simulink model "Lab2Videoblock"  (R2022a)
settings: Solver=VariableStepAuto  StartTime=0.0  StopTime=1  MaxStep=1e-4  RelTol=1e-3
undefined symbols (not defined in the file or in its folder): ACsource, Angle, DCsource, load, transparam
libraries: spsFourierLib x4, spsGroundLib x4, spsVoltageMeasurementLib x4, spsCurrentMeasurementLib x3, spsACVoltageSourceLib x1, spsDiodeLib x1, spsDCVoltageSourceLib x1, spsLinearTransformerLib x1, spsMultimeterLib x1, spsSeriesRLCBranchLib x1, spsRMSLib x1, spsUniversalBridgeLib x1
settings Model: Creator=Student11  LastModifiedBy=админ
settings SolverCC: AlgebraicLoopSolver=TrustRegion
settings DataIOCC: ReturnWorkspaceOutputs=off
settings DebuggingCC: SFMachineParentedDataDiag=warning  ArithmeticOperatorsInVariantConditions=warning
settings SFSimCC: SimUseLocalCustomCode=off  CustomCodeUndefinedFunction=UseInterfaceOnly
settings RTWCC: RTWUseLocalCustomCode=off
settings CodeAppCC: StateflowObjectComments=on
settings SimscapeCC: SimscapeNormalizeSystem=off

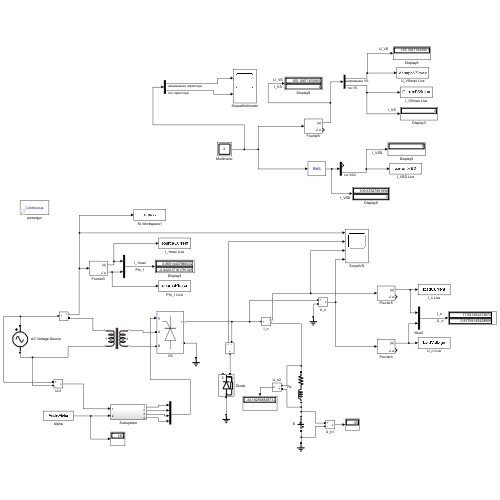
[thumbnail: Simulink's stored preview of the top-level diagram]
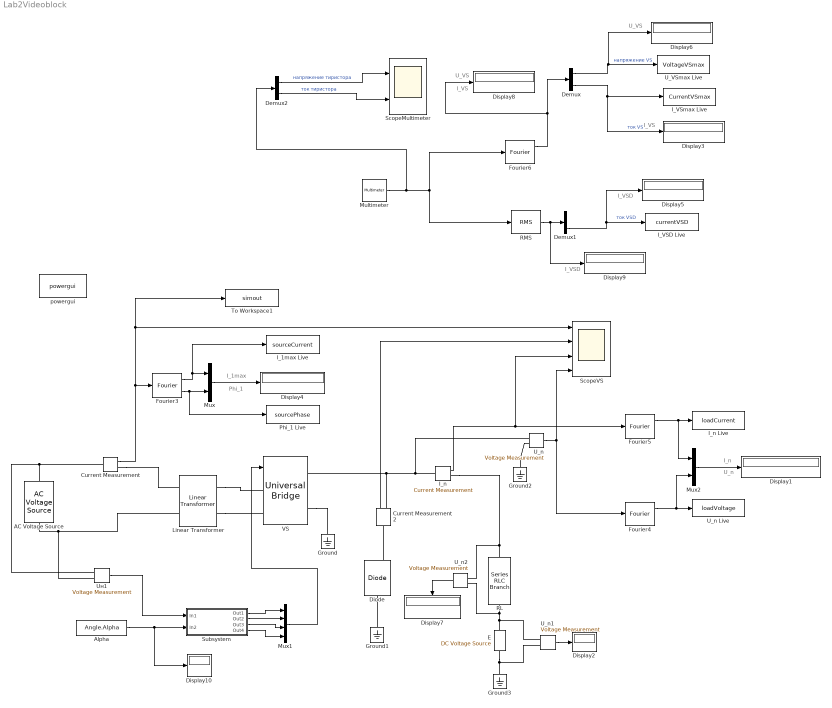
== system Lab2Videoblock ==
  note: U_VS
  note: I_VS
  note: I_VSD
  note: Phi_1
  note: I_1max
  note: I_n
  note: U_n
  note: I_VS
  note: U_VS
  note: I_VSD
  AC Voltage Source : spsACVoltageSourceLib/AC Voltage Source  Amplitude=ACsource.voltage  Phase=0  Frequency=ACsource.freq  SampleTime=0  Measurements=None  BusType=swing  Pref=10e3  Qref=0  Qmin=-inf  Qmax=+inf
  Alpha : Constant  Value=Angle.Alpha
  Current Measurement : spsCurrentMeasurementLib/Current Measurement  PhasorSimulation=off  OutputType=Complex  PSBequivalent=0
  Current Measurement2 : spsCurrentMeasurementLib/Current Measurement  PhasorSimulation=off  OutputType=Complex  PSBequivalent=0
  Demux : Demux  Outputs=2
  Demux1 : Demux  Outputs=2
  Demux2 : Demux  Outputs=2
  Diode : spsDiodeLib/Diode  Ron=0.001  Lon=0  Vf=0.8  IC=0  UseSnubber=0  Rs=500  Cs=250e-9  Measurements=on
  Display{1..10} (10 alike) : Display
      Display1 settings: Format=binary (Stored Integer)
      Display10 settings: Format=binary (Stored Integer)
      Display2 settings: Format=binary (Stored Integer)
      Display3 settings: Format=binary (Stored Integer)  Decimation=2
      Display4 settings: Format=binary (Stored Integer)  Decimation=2
      Display5 settings: Format=binary (Stored Integer)  Decimation=2
      Display6 settings: Format=binary (Stored Integer)  Decimation=2
      Display7 settings: Format=binary (Stored Integer)
      Display8 settings: Format=binary (Stored Integer)  Decimation=2
      Display9 settings: Format=binary (Stored Integer)  Decimation=2
  E : spsDCVoltageSourceLib/DC Voltage Source  Amplitude=DCsource.voltage  Measurements=None
  Fourier3 : spsFourierLib/Fourier  Freq=ACsource.freq  n=1  InInit=[0, 0]  Ts=0
      settings: SourceProductBaseCode=PS
  Fourier4 : spsFourierLib/Fourier  Freq=ACsource.freq  n=0  InInit=[0, 0]  Ts=0
      settings: SourceProductBaseCode=PS
  Fourier5 : spsFourierLib/Fourier  Freq=ACsource.freq  n=0  InInit=[0, 0]  Ts=0
      settings: SourceProductBaseCode=PS
  Fourier6 : spsFourierLib/Fourier  Freq=ACsource.freq  n=1  InInit=[0, 0]  Ts=0
      settings: SourceProductBaseCode=PS
  Ground{,1..3} (4 alike) : spsGroundLib/Ground  LConnTagsString=a
  I_1max Live : ToWorkspace  VariableName=sourceCurrent  SampleTime=0.0002
      settings: Save2DSignal=2-D array (concatenate along first dimension)
  I_VSD Live : ToWorkspace  VariableName=currentVSD  SampleTime=0.0002
      settings: Save2DSignal=2-D array (concatenate along first dimension)
  I_VSmax Live : ToWorkspace  VariableName=CurrentVSmax  SampleTime=-1
      settings: Save2DSignal=2-D array (concatenate along first dimension)
  I_n : spsCurrentMeasurementLib/Current Measurement  PhasorSimulation=off  OutputType=Complex  PSBequivalent=0
  I_n Live : ToWorkspace  VariableName=loadCurrent  SampleTime=-1
      settings: Save2DSignal=2-D array (concatenate along first dimension)
  Linear Transformer : spsLinearTransformerLib/Linear Transformer  UNITS=SI  NominalPower=[transparam.power ACsource.freq]  winding1=[transparam.volt1wing 0.01 0.000001]  winding2=[transparam.volt2wing 0.04 0.000004]  ThreeWindings=off  winding3=[3.15e+05 992.25 63.169]  RmLm=[5000 5000]  Measurements=None  DataType=on
  Multimeter : spsMultimeterLib/Multimeter  L=10  sel=[1 7]  yselected={}  Gain=[1 1]  OutputType=Complex  PlotAtSimulationStop=off  PhasorSimulation=off
  Mux : Mux  Inputs=2
  Mux1 : Mux
  Mux2 : Mux  Inputs=2
  Phi_1 Live : ToWorkspace  VariableName=sourcePhase  SampleTime=0.0002
      settings: Save2DSignal=2-D array (concatenate along first dimension)
  RL : spsSeriesRLCBranchLib/Series RLC Branch  LConnTagsString=__new0  RConnTagsString=__new0  BranchType=RL  Resistance=load.Res  Inductance=load.Ind  SetiL0=off  InitialCurrent=0  Capacitance=1e-6  Setx0=off  InitialVoltage=0  Measurements=None
  RMS : spsRMSLib/RMS  TrueRMS=on  Freq=ACsource.freq  RMSInit=0  Ts=0
  ScopeMultimeter : Scope  NumInputPorts=2
  ScopeVS : Scope  NumInputPorts=4
  Subsystem : Subsystem
  To Workspace1 : ToWorkspace  VariableName=simout  SampleTime=0.0002
      settings: Save2DSignal=2-D array (concatenate along first dimension)
  U_VSmax Live : ToWorkspace  VariableName=VoltageVSmax  SampleTime=-1
      settings: Save2DSignal=2-D array (concatenate along first dimension)
  U_n : spsVoltageMeasurementLib/Voltage Measurement  PhasorSimulation=off  OutputType=Complex  PSBequivalent=0
  U_n Live : ToWorkspace  VariableName=loadVoltage  SampleTime=0.0002
      settings: Save2DSignal=2-D array (concatenate along first dimension)
  U_n1 : spsVoltageMeasurementLib/Voltage Measurement  PhasorSimulation=off  OutputType=Complex  PSBequivalent=0
  U_n2 : spsVoltageMeasurementLib/Voltage Measurement  PhasorSimulation=off  OutputType=Complex  PSBequivalent=0
  Uн1 : spsVoltageMeasurementLib/Voltage Measurement  PhasorSimulation=off  OutputType=Complex  PSBequivalent=0
  VS : spsUniversalBridgeLib/Universal Bridge  Arms=2  SnubberResistance=1e5  SnubberCapacitance=1e-6  Device=Thyristors  Ron=1e-3  Lon=0  ForwardVoltages="[  0  0  ]"  ForwardVoltage=2  GTOparameters=[ 10e-6 , 20e-6 ]  IGBTparameters=[ 1e-6 , 2e-6 ]  Measurements=All voltages and currents  Measurements_2=None  converterType=Rectifier
  powergui : spspowerguiLib/powergui  Priority=1  SimulationMode=Continuous  SampleTime=50e-6  frequency=60  Iterations=50  frequencyindice=0  Pbase=100e6  ErrMax=1e-4  UnitsV=kV  UnitsW=MW  buscounter=0  FunctionMessages=off  echomessages=off  EnableUseOfTLC=off  CurrentSourceSwitches=off  DisableSnubberDevices=off  DisableRonSwitches=off  DisableVfSwitches=off  DisplayEquations=off  AutomaticDiscreteSolvers=off  SolverType=Tustin/Backward Euler (TBE)  Interpol=off  ExternalGateDelay=off  methode=off  Ts=100  x0status=blocks  SPID=on  SwTol=0  HookPort=off  NonlinearTolerance=1e-4  nMaxIteration=100  ContinueOnMaxIteration=off  RestoreLinks=warning  ResistiveCurrentMeasurement=off  Frange=[0:2:500]  Ylog=off  Xlog=on  ShowGrid=off  save=off  variable=ZData  structure=0  ZoomFFT=off  StartTime=0.0  cycles=1  DisplayStyle=1  fundamental=60  FreqAxis=off  MaxFrequency=1000  frequencyindicesteady=1  RmsSteady=1  display=off
  wires:
  Alpha/1 -> Display10/1, Subsystem/2(In2)
  Uн1/1 -> Subsystem/1(In1)
  Current Measurement/1 -> ScopeVS/1, To Workspace1/1, Fourier3/1
  Fourier3/2 -> Phi_1 Live/1, Mux/2
  Fourier3/1 -> I_1max Live/1, Mux/1
  Mux/1 -> Display4/1
  Subsystem/4(Out4) -> Mux1/4
  Subsystem/3(Out3) -> Mux1/3
  Subsystem/2(Out2) -> Mux1/2
  Subsystem/1(Out1) -> Mux1/1
  Mux1/1 -> VS/1
  Current Measurement2/1 -> ScopeVS/2
  U_n/1 -> ScopeVS/4, Fourier4/1
  I_n/1 -> ScopeVS/3, Fourier5/1
  Mux2/1 -> Display1/1
  Multimeter/1 -> Demux2/1, RMS/1, Fourier6/1
  Fourier6/1 -> Demux/1, Display8/1
  Demux/1 -> Display6/1, U_VSmax Live/1  "напряжение VS"
  Demux/2 -> Display3/1, I_VSmax Live/1  "ток VS"
  RMS/1 -> Display9/1, Demux1/1
  Demux1/2 -> Display5/1, I_VSD Live/1  "ток VSD"
  U_n2/1 -> Display7/1
  Fourier5/1 -> Mux2/1, I_n Live/1
  Fourier4/1 -> U_n Live/1, Mux2/2
  Demux2/1 -> ScopeMultimeter/1  "напряжение тиристора"
  Demux2/2 -> ScopeMultimeter/2  "ток тиристора"
  U_n1/1 -> Display2/1
  connections:
  Current Measurement/RConn1 -- Linear Transformer/LConn1
  AC Voltage Source/RConn1 -- Current Measurement/LConn1 -- Uн1/LConn1
  Linear Transformer/LConn2 -- Uн1/LConn2 -- AC Voltage Source/LConn1
  Linear Transformer/RConn1 -- VS/LConn1
  Linear Transformer/RConn2 -- VS/LConn2
  VS/RConn2 -- Ground/LConn1
  I_n/LConn1 -- Current Measurement2/RConn1 -- VS/RConn1 -- U_n/LConn1
  Diode/RConn1 -- Current Measurement2/LConn1
  Ground1/LConn1 -- Diode/LConn1
  I_n/RConn1 -- U_n2/LConn2 -- RL/LConn1
  U_n1/LConn1 -- U_n2/LConn1 -- RL/RConn1 -- E/LConn1
  U_n1/LConn2 -- E/RConn1 -- Ground3/LConn1
  Ground2/LConn1 -- U_n/LConn2

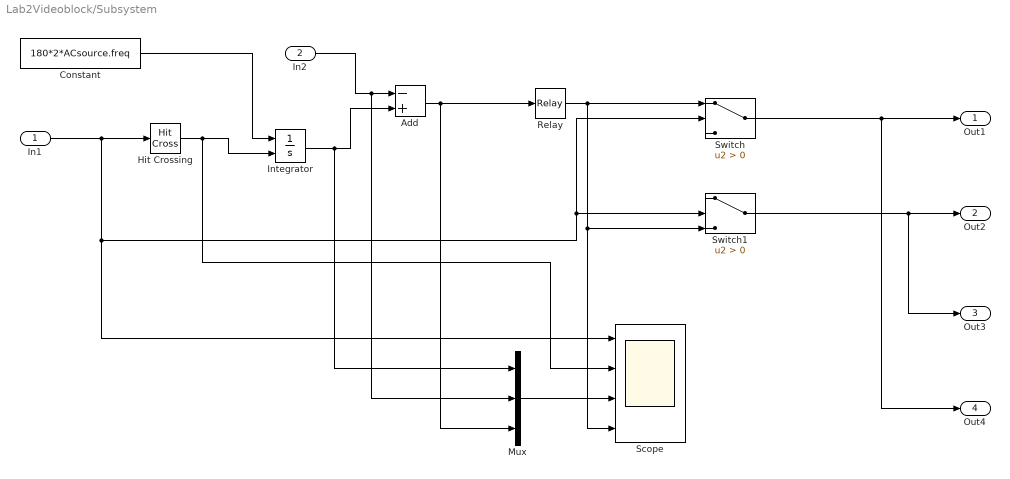
== system Lab2Videoblock/Subsystem ==
  In1 : Inport
  In2 : Inport  Port=2
  Add : Sum  Inputs=-+
  Constant : Constant  Value=180*2*ACsource.freq
  Hit Crossing : HitCross
  Integrator : Integrator  ExternalReset=rising
  Mux : Mux  Inputs=3
  Relay : Relay  OffSwitchValue=0
  Scope : Scope  NumInputPorts=4
  Switch : Switch  Criteria=u2 > Threshold  SaturateOnIntegerOverflow=off  InputSameDT=off
  Switch1 : Switch  Criteria=u2 > Threshold  SaturateOnIntegerOverflow=off  InputSameDT=off
  Out1 : Outport
  Out2 : Outport  Port=2
  Out3 : Outport  Port=3
  Out4 : Outport  Port=4
  wires:
  In2/1 -> Mux/2, Add/1
  Hit Crossing/1 -> Scope/2, Integrator/2
  Constant/1 -> Integrator/1
  Add/1 -> Mux/3, Relay/1
  Relay/1 -> Switch1/3, Scope/4, Switch/1
  Switch1/1 -> Out3/1, Out2/1
  Switch/1 -> Out4/1, Out1/1
  In1/1 -> Switch1/2, Switch/2, Scope/1, Hit Crossing/1
  Mux/1 -> Scope/3
  Integrator/1 -> Mux/1, Add/2
